simulink model "Problem_4"  (R2020a)
settings: Solver=VariableStepAuto  StartTime=0.0  StopTime=10.0  RelTol=1e-3
settings Model: Creator=USER  LastModifiedBy=USER

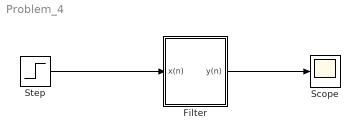
== system Problem_4 ==
  Filter : Subsystem
  Scope : Scope
  Step : Step  SampleTime=0
  wires:
  Step/1 -> Filter/1(x(n))
  Filter/1(y(n)) -> Scope/1

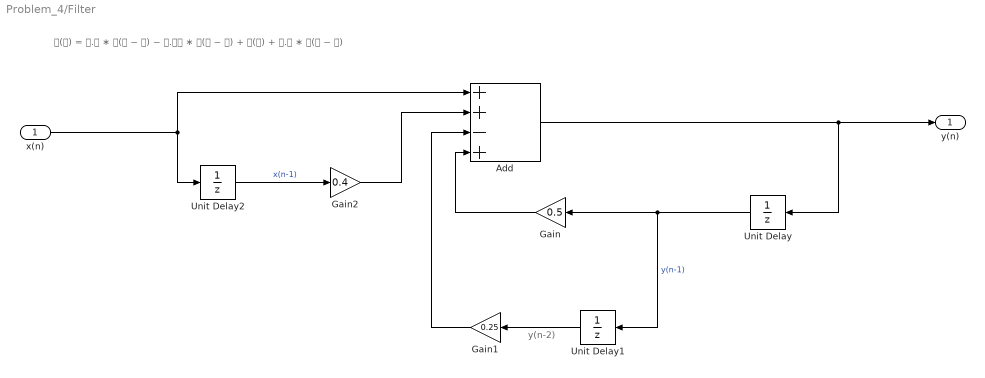
== system Problem_4/Filter ==
  note: y(n-2)
  note: 𝐲(𝐧) = 𝟎.𝟓 ∗ 𝐲(𝐧 − 𝟏) − 𝟎.𝟐𝟓 ∗ 𝐲(𝐧 − 𝟐) + 𝐱(𝐧) + 𝟎.𝟒 ∗ 𝐱(𝐧 − 𝟏)
  x(n) : Inport
  Add : Sum  Inputs=++-+
  Gain : Gain  Gain=0.5
  Gain1 : Gain  Gain=0.25
  Gain2 : Gain  Gain=0.4
  Unit Delay : UnitDelay  SampleTime=-1  HasFrameUpgradeWarning=on
  Unit Delay1 : UnitDelay  SampleTime=-1  HasFrameUpgradeWarning=on
  Unit Delay2 : UnitDelay  SampleTime=-1  HasFrameUpgradeWarning=on
  y(n) : Outport
  wires:
  Add/1 -> y(n)/1, Unit Delay/1
  Unit Delay1/1 -> Gain1/1
  Gain/1 -> Add/4
  x(n)/1 -> Unit Delay2/1, Add/1
  Unit Delay2/1 -> Gain2/1  "x(n-1)"
  Gain1/1 -> Add/3
  Unit Delay/1 -> Unit Delay1/1, Gain/1  "y(n-1)"
  Gain2/1 -> Add/2
